simulink model "Casc_Filter_x4"  (Simulink 6.4)
settings: Solver=ode45  StartTime=0.0  StopTime=4100/sampling_freq  RelTol=1e-3
undefined symbols (not defined in the file): A, B, filter_clk, Fs, get, h_g, h_k, PCIN, sampling_freq
libraries: xbsIndex_r4 x851, dspsnks4 x9, simulink x2, dspsrcs4 x1
(part 1 of 8)
settings Model: LastModifiedBy=tbrimeye

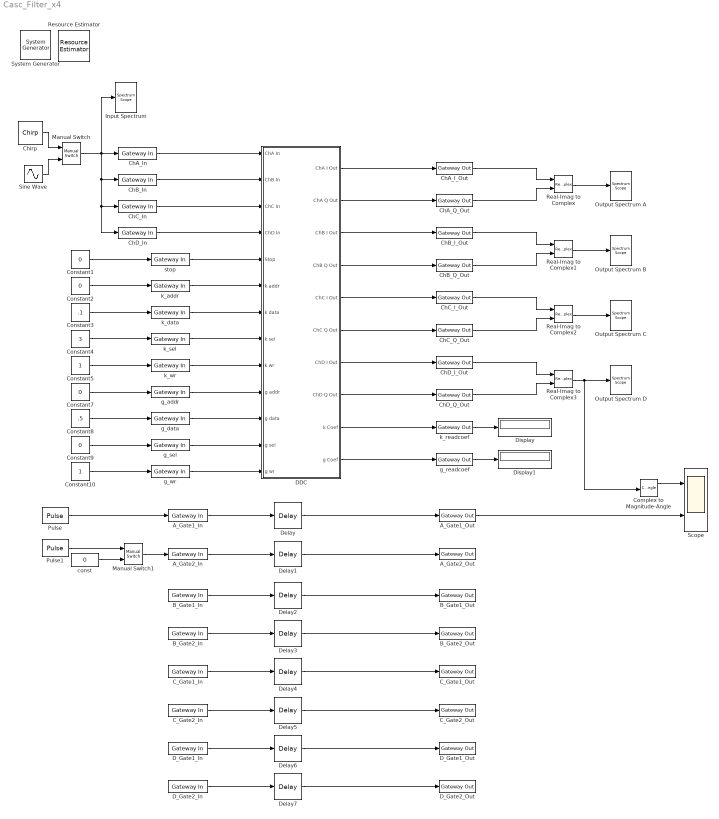
== system Casc_Filter_x4 ==
  " System Generator" : xbsIndex_r4/ System Generator  Tag=genX  SystemSampleTime=-1  xilinxfamily=Virtex4  part=xc4vsx35  speed=-11  package=ff668  synthesis_tool=XST  directory=C:/Work_Projects/Xilinx/SysGen_Outputs/DDC_Filters/Casc_Filter_x4_netlist  testbench=off  simulink_period=1/filter_clk  sysclk_period=(1/filter_clk)*1e9  incr_netlist=off  trim_vbits=Everywhere in SubSystem  dbl_ovrd=According to Block Masks  core_generation=According to Block Masks  run_coregen=off  deprecated_control=off  eval_field=0  block_type=sysgen
      settings: block_version=8.2
  A_Gate1_In : xbsIndex_r4/Gateway In  arith_type=Boolean  n_bits=18  bin_pt=0  quantization="Round  (unbiased: +/- Inf)"  overflow=Flag as error  period=1/12e6  dbl_ovrd=off  timing_constraint=None  locs_specified=off  LOCs={}  block_type=gatewayin
      settings: infoedit="Gateway in block.  Converts inputs of type Simulink integer, double and fixed point to  Xilinx fixed point type.<P><P>Hardware notes:  In hardware these blocks become top level input ports."  xl_area=[0 0 0 0 1 0 0]  block_version=8.2
  A_Gate1_Out : xbsIndex_r4/Gateway Out  hdl_port=on  timing_constraint=None  locs_specified=off  LOCs={}  block_type=gatewayout
      settings: infoedit="Gateway out block.  Converts Xilinx fixed point inputs into ouputs of type Simulink integer, double, or fixed point.<P><P>Hardware notes:  In hardware these blocks become top level output ports or are discarded, depending on how they are configured."  xl_area=[0 0 0 0 18 0 0]  block_version=VER_STRING_GOES_HERE
  A_Gate2_In : xbsIndex_r4/Gateway In  arith_type=Boolean  n_bits=18  bin_pt=0  quantization="Round  (unbiased: +/- Inf)"  overflow=Flag as error  period=1/12e6  dbl_ovrd=off  timing_constraint=None  locs_specified=off  LOCs={}  block_type=gatewayin
      settings: infoedit="Gateway in block.  Converts inputs of type Simulink integer, double and fixed point to  Xilinx fixed point type.<P><P>Hardware notes:  In hardware these blocks become top level input ports."  xl_area=[0 0 0 0 1 0 0]  block_version=8.2
  A_Gate2_Out : xbsIndex_r4/Gateway Out  hdl_port=on  timing_constraint=None  locs_specified=off  LOCs={}  block_type=gatewayout
      settings: infoedit="Gateway out block.  Converts Xilinx fixed point inputs into ouputs of type Simulink integer, double, or fixed point.<P><P>Hardware notes:  In hardware these blocks become top level output ports or are discarded, depending on how they are configured."  xl_area=[0 0 0 0 18 0 0]  block_version=VER_STRING_GOES_HERE
  B_Gate1_In : xbsIndex_r4/Gateway In  arith_type=Boolean  n_bits=18  bin_pt=0  quantization="Round  (unbiased: +/- Inf)"  overflow=Flag as error  period=1/12e6  dbl_ovrd=off  timing_constraint=None  locs_specified=off  LOCs={}  block_type=gatewayin
      settings: infoedit="Gateway in block.  Converts inputs of type Simulink integer, double and fixed point to  Xilinx fixed point type.<P><P>Hardware notes:  In hardware these blocks become top level input ports."  xl_area=[0 0 0 0 1 0 0]  block_version=8.2
  B_Gate1_Out : xbsIndex_r4/Gateway Out  hdl_port=on  timing_constraint=None  locs_specified=off  LOCs={}  block_type=gatewayout
      settings: infoedit="Gateway out block.  Converts Xilinx fixed point inputs into ouputs of type Simulink integer, double, or fixed point.<P><P>Hardware notes:  In hardware these blocks become top level output ports or are discarded, depending on how they are configured."  xl_area=[0 0 0 0 18 0 0]  block_version=VER_STRING_GOES_HERE
  B_Gate2_In : xbsIndex_r4/Gateway In  arith_type=Boolean  n_bits=18  bin_pt=0  quantization="Round  (unbiased: +/- Inf)"  overflow=Flag as error  period=1/12e6  dbl_ovrd=off  timing_constraint=None  locs_specified=off  LOCs={}  block_type=gatewayin
      settings: infoedit="Gateway in block.  Converts inputs of type Simulink integer, double and fixed point to  Xilinx fixed point type.<P><P>Hardware notes:  In hardware these blocks become top level input ports."  xl_area=[0 0 0 0 1 0 0]  block_version=8.2
  B_Gate2_Out : xbsIndex_r4/Gateway Out  hdl_port=on  timing_constraint=None  locs_specified=off  LOCs={}  block_type=gatewayout
      settings: infoedit="Gateway out block.  Converts Xilinx fixed point inputs into ouputs of type Simulink integer, double, or fixed point.<P><P>Hardware notes:  In hardware these blocks become top level output ports or are discarded, depending on how they are configured."  xl_area=[0 0 0 0 18 0 0]  block_version=VER_STRING_GOES_HERE
  C_Gate1_In : xbsIndex_r4/Gateway In  arith_type=Boolean  n_bits=18  bin_pt=0  quantization="Round  (unbiased: +/- Inf)"  overflow=Flag as error  period=1/12e6  dbl_ovrd=off  timing_constraint=None  locs_specified=off  LOCs={}  block_type=gatewayin
      settings: infoedit="Gateway in block.  Converts inputs of type Simulink integer, double and fixed point to  Xilinx fixed point type.<P><P>Hardware notes:  In hardware these blocks become top level input ports."  xl_area=[0 0 0 0 1 0 0]  block_version=8.2
  C_Gate1_Out : xbsIndex_r4/Gateway Out  hdl_port=on  timing_constraint=None  locs_specified=off  LOCs={}  block_type=gatewayout
      settings: infoedit="Gateway out block.  Converts Xilinx fixed point inputs into ouputs of type Simulink integer, double, or fixed point.<P><P>Hardware notes:  In hardware these blocks become top level output ports or are discarded, depending on how they are configured."  xl_area=[0 0 0 0 18 0 0]  block_version=VER_STRING_GOES_HERE
  C_Gate2_In : xbsIndex_r4/Gateway In  arith_type=Boolean  n_bits=18  bin_pt=0  quantization="Round  (unbiased: +/- Inf)"  overflow=Flag as error  period=1/12e6  dbl_ovrd=off  timing_constraint=None  locs_specified=off  LOCs={}  block_type=gatewayin
      settings: infoedit="Gateway in block.  Converts inputs of type Simulink integer, double and fixed point to  Xilinx fixed point type.<P><P>Hardware notes:  In hardware these blocks become top level input ports."  xl_area=[0 0 0 0 1 0 0]  block_version=8.2
  C_Gate2_Out : xbsIndex_r4/Gateway Out  hdl_port=on  timing_constraint=None  locs_specified=off  LOCs={}  block_type=gatewayout
      settings: infoedit="Gateway out block.  Converts Xilinx fixed point inputs into ouputs of type Simulink integer, double, or fixed point.<P><P>Hardware notes:  In hardware these blocks become top level output ports or are discarded, depending on how they are configured."  xl_area=[0 0 0 0 18 0 0]  block_version=VER_STRING_GOES_HERE
  ChA_I_Out : xbsIndex_r4/Gateway Out  hdl_port=on  timing_constraint=None  locs_specified=off  LOCs={}  block_type=gatewayout
      settings: infoedit="Gateway out block.  Converts Xilinx fixed point inputs into ouputs of type Simulink integer, double, or fixed point.<P><P>Hardware notes:  In hardware these blocks become top level output ports or are discarded, depending on how they are configured."  xl_area=[0 0 0 0 16 0 0]  block_version=8.2
  ChA_In : xbsIndex_r4/Gateway In  arith_type="Signed  (2's comp)"  n_bits=14  bin_pt=13  quantization="Round  (unbiased: +/- Inf)"  overflow=Saturate  period=1/sampling_freq  dbl_ovrd=off  timing_constraint=None  locs_specified=off  LOCs={}  block_type=gatewayin
      settings: infoedit="Gateway in block.  Converts inputs of type Simulink integer, double and fixed point to  Xilinx fixed point type.<P><P>Hardware notes:  In hardware these blocks become top level input ports."  xl_area=[0 0 0 0 14 0 0]  block_version=8.2
  ChA_Q_Out : xbsIndex_r4/Gateway Out  hdl_port=on  timing_constraint=None  locs_specified=off  LOCs={}  block_type=gatewayout
      settings: infoedit="Gateway out block.  Converts Xilinx fixed point inputs into ouputs of type Simulink integer, double, or fixed point.<P><P>Hardware notes:  In hardware these blocks become top level output ports or are discarded, depending on how they are configured."  xl_area=[0 0 0 0 16 0 0]  block_version=8.2
  ChB_I_Out : xbsIndex_r4/Gateway Out  hdl_port=on  timing_constraint=None  locs_specified=off  LOCs={}  block_type=gatewayout
      settings: infoedit="Gateway out block.  Converts Xilinx fixed point inputs into ouputs of type Simulink integer, double, or fixed point.<P><P>Hardware notes:  In hardware these blocks become top level output ports or are discarded, depending on how they are configured."  xl_area=[0 0 0 0 16 0 0]  block_version=8.2
  ChB_In : xbsIndex_r4/Gateway In  arith_type="Signed  (2's comp)"  n_bits=14  bin_pt=13  quantization="Round  (unbiased: +/- Inf)"  overflow=Saturate  period=1/sampling_freq  dbl_ovrd=off  timing_constraint=None  locs_specified=off  LOCs={}  block_type=gatewayin
      settings: infoedit="Gateway in block.  Converts inputs of type Simulink integer, double and fixed point to  Xilinx fixed point type.<P><P>Hardware notes:  In hardware these blocks become top level input ports."  xl_area=[0 0 0 0 14 0 0]  block_version=8.2
  ChB_Q_Out : xbsIndex_r4/Gateway Out  hdl_port=on  timing_constraint=None  locs_specified=off  LOCs={}  block_type=gatewayout
      settings: infoedit="Gateway out block.  Converts Xilinx fixed point inputs into ouputs of type Simulink integer, double, or fixed point.<P><P>Hardware notes:  In hardware these blocks become top level output ports or are discarded, depending on how they are configured."  xl_area=[0 0 0 0 16 0 0]  block_version=8.2
  ChC_I_Out : xbsIndex_r4/Gateway Out  hdl_port=on  timing_constraint=None  locs_specified=off  LOCs={}  block_type=gatewayout
      settings: infoedit="Gateway out block.  Converts Xilinx fixed point inputs into ouputs of type Simulink integer, double, or fixed point.<P><P>Hardware notes:  In hardware these blocks become top level output ports or are discarded, depending on how they are configured."  xl_area=[0 0 0 0 16 0 0]  block_version=8.2
  ChC_In : xbsIndex_r4/Gateway In  arith_type="Signed  (2's comp)"  n_bits=14  bin_pt=13  quantization="Round  (unbiased: +/- Inf)"  overflow=Saturate  period=1/sampling_freq  dbl_ovrd=off  timing_constraint=None  locs_specified=off  LOCs={}  block_type=gatewayin
      settings: infoedit="Gateway in block.  Converts inputs of type Simulink integer, double and fixed point to  Xilinx fixed point type.<P><P>Hardware notes:  In hardware these blocks become top level input ports."  xl_area=[0 0 0 0 14 0 0]  block_version=8.2
  ChC_Q_Out : xbsIndex_r4/Gateway Out  hdl_port=on  timing_constraint=None  locs_specified=off  LOCs={}  block_type=gatewayout
      settings: infoedit="Gateway out block.  Converts Xilinx fixed point inputs into ouputs of type Simulink integer, double, or fixed point.<P><P>Hardware notes:  In hardware these blocks become top level output ports or are discarded, depending on how they are configured."  xl_area=[0 0 0 0 16 0 0]  block_version=8.2
  ChD_I_Out : xbsIndex_r4/Gateway Out  hdl_port=on  timing_constraint=None  locs_specified=off  LOCs={}  block_type=gatewayout
      settings: infoedit="Gateway out block.  Converts Xilinx fixed point inputs into ouputs of type Simulink integer, double, or fixed point.<P><P>Hardware notes:  In hardware these blocks become top level output ports or are discarded, depending on how they are configured."  xl_area=[0 0 0 0 16 0 0]  block_version=8.2
  ChD_In : xbsIndex_r4/Gateway In  arith_type="Signed  (2's comp)"  n_bits=14  bin_pt=13  quantization="Round  (unbiased: +/- Inf)"  overflow=Saturate  period=1/sampling_freq  dbl_ovrd=off  timing_constraint=None  locs_specified=off  LOCs={}  block_type=gatewayin
      settings: infoedit="Gateway in block.  Converts inputs of type Simulink integer, double and fixed point to  Xilinx fixed point type.<P><P>Hardware notes:  In hardware these blocks become top level input ports."  xl_area=[0 0 0 0 14 0 0]  block_version=8.2
  ChD_Q_Out : xbsIndex_r4/Gateway Out  hdl_port=on  timing_constraint=None  locs_specified=off  LOCs={}  block_type=gatewayout
      settings: infoedit="Gateway out block.  Converts Xilinx fixed point inputs into ouputs of type Simulink integer, double, or fixed point.<P><P>Hardware notes:  In hardware these blocks become top level output ports or are discarded, depending on how they are configured."  xl_area=[0 0 0 0 16 0 0]  block_version=8.2
  Chirp : dspsrcs4/Chirp  sweep=Linear  mode=Unidirectional  f0=0  f1=sampling_freq_div2  t1=4096/sampling_freq  Tsweep=4096/sampling_freq  phase=pi/4  Ts=1/sampling_freq  spf=1  datatype=Double
  Complex to Magnitude-Angle : ComplexToMagnitudeAngle
  Constant{1..2,7,9} (4 alike) : Constant  Value=0  OutDataType=sfix(16)  ConRadixGroup=Use specified scaling  OutScaling=2^0  SampleTime=inf  FramePeriod=inf
  Constant10 : Constant  Value=1  OutDataType=sfix(16)  ConRadixGroup=Use specified scaling  OutScaling=2^0  SampleTime=inf  FramePeriod=inf
  Constant3 : Constant  Value=.1  OutDataType=sfix(16)  ConRadixGroup=Use specified scaling  OutScaling=2^0  SampleTime=inf  FramePeriod=inf
  Constant4 : Constant  Value=3  OutDataType=sfix(16)  ConRadixGroup=Use specified scaling  OutScaling=2^0  SampleTime=inf  FramePeriod=inf
  Constant5 : Constant  Value=1  OutDataType=sfix(16)  ConRadixGroup=Use specified scaling  OutScaling=2^0  SampleTime=inf  FramePeriod=inf
  Constant8 : Constant  Value=.5  OutDataType=sfix(16)  ConRadixGroup=Use specified scaling  OutScaling=2^0  SampleTime=inf  FramePeriod=inf
  DDC : Subsystem
  D_Gate1_In : xbsIndex_r4/Gateway In  arith_type=Boolean  n_bits=18  bin_pt=0  quantization="Round  (unbiased: +/- Inf)"  overflow=Flag as error  period=1/12e6  dbl_ovrd=off  timing_constraint=None  locs_specified=off  LOCs={}  block_type=gatewayin
      settings: infoedit="Gateway in block.  Converts inputs of type Simulink integer, double and fixed point to  Xilinx fixed point type.<P><P>Hardware notes:  In hardware these blocks become top level input ports."  xl_area=[0 0 0 0 1 0 0]  block_version=8.2
  D_Gate1_Out : xbsIndex_r4/Gateway Out  hdl_port=on  timing_constraint=None  locs_specified=off  LOCs={}  block_type=gatewayout
      settings: infoedit="Gateway out block.  Converts Xilinx fixed point inputs into ouputs of type Simulink integer, double, or fixed point.<P><P>Hardware notes:  In hardware these blocks become top level output ports or are discarded, depending on how they are configured."  xl_area=[0 0 0 0 18 0 0]  block_version=VER_STRING_GOES_HERE
  D_Gate2_In : xbsIndex_r4/Gateway In  arith_type=Boolean  n_bits=18  bin_pt=0  quantization="Round  (unbiased: +/- Inf)"  overflow=Flag as error  period=1/12e6  dbl_ovrd=off  timing_constraint=None  locs_specified=off  LOCs={}  block_type=gatewayin
      settings: infoedit="Gateway in block.  Converts inputs of type Simulink integer, double and fixed point to  Xilinx fixed point type.<P><P>Hardware notes:  In hardware these blocks become top level input ports."  xl_area=[0 0 0 0 1 0 0]  block_version=8.2
  D_Gate2_Out : xbsIndex_r4/Gateway Out  hdl_port=on  timing_constraint=None  locs_specified=off  LOCs={}  block_type=gatewayout
      settings: infoedit="Gateway out block.  Converts Xilinx fixed point inputs into ouputs of type Simulink integer, double, or fixed point.<P><P>Hardware notes:  In hardware these blocks become top level output ports or are discarded, depending on how they are configured."  xl_area=[0 0 0 0 18 0 0]  block_version=VER_STRING_GOES_HERE
  Delay{,1..7} (8 alike) : xbsIndex_r4/Delay  en=off  latency=9  dbl_ovrd=off  reg_retiming=off  block_type=delay
      settings: infoedit=Hardware notes: A delay line is a chain, each link of which is an SRL16 followed by a flip-flop. If register retiming is enabled, the delay line is a chain of flip-flops.  block_version=8.2
  Display : Display
  Display1 : Display
  Input Spectrum : dspsnks4/Spectrum Scope  DialogController=dspdialog.SpectrumScope  DialogControllerArgs=DataTag5  SystemSampleTime=-1  ScopeProperties=on  Domain=Frequency  HorizSpan=1  UseBuffer=on  BufferSize=4096  Overlap=64  inpFftLenInherit=on  FFTlength=4096  numAvg=2  DisplayProperties=off  AxisGrid=on  Memory=off  FrameNumber=on  AxisLegend=off  AxisZoom=off  OpenScopeAtSimStart=on  OpenScopeImmediately=off  FigPos=get(0,'defaultfigureposition')  AxisProperties=off  XUnits=Hertz  XRange=[-Fs/2...Fs/2]  InheritXIncr=on  XIncr=1.0  XLabel=Samples  YUnits=dB  YLabel=Magnitude-squared, dB  LineProperties=off  wintypeSpecScope=Boxcar  RsSpecScope=50  betaSpecScope=5  winsampSpecScope=Periodic
      settings: YMin=-100  YMax=0
  Manual Switch : simulink/Signal Routing/Manual Switch  SystemSampleTime=-1  sw=1  action=0
  Manual Switch1 : simulink/Signal Routing/Manual Switch  SystemSampleTime=-1  sw=0  action=0
  Output Spectrum A : dspsnks4/Spectrum Scope  DialogController=dspdialog.SpectrumScope  DialogControllerArgs=DataTag6  SystemSampleTime=-1  ScopeProperties=on  Domain=Frequency  HorizSpan=1  UseBuffer=on  BufferSize=1024  Overlap=64  inpFftLenInherit=on  FFTlength=1024  numAvg=2  DisplayProperties=off  AxisGrid=on  Memory=off  FrameNumber=on  AxisLegend=off  AxisZoom=off  OpenScopeAtSimStart=on  OpenScopeImmediately=off  FigPos=get(0,'defaultfigureposition')  AxisProperties=off  XUnits=Hertz  XRange=[-Fs/2...Fs/2]  InheritXIncr=on  XIncr=1.0  XLabel=Samples  YUnits=dB  YLabel=Magnitude-squared, dB  LineProperties=off  wintypeSpecScope=Boxcar  RsSpecScope=50  betaSpecScope=5  winsampSpecScope=Periodic
      settings: YMin=-120  YMax=0
  Output Spectrum B : dspsnks4/Spectrum Scope  DialogController=dspdialog.SpectrumScope  DialogControllerArgs=DataTag7  SystemSampleTime=-1  ScopeProperties=on  Domain=Frequency  HorizSpan=1  UseBuffer=on  BufferSize=1024  Overlap=64  inpFftLenInherit=on  FFTlength=1024  numAvg=2  DisplayProperties=off  AxisGrid=on  Memory=off  FrameNumber=on  AxisLegend=off  AxisZoom=off  OpenScopeAtSimStart=on  OpenScopeImmediately=off  FigPos=get(0,'defaultfigureposition')  AxisProperties=off  XUnits=Hertz  XRange=[-Fs/2...Fs/2]  InheritXIncr=on  XIncr=1.0  XLabel=Samples  YUnits=dB  YLabel=Magnitude-squared, dB  LineProperties=off  wintypeSpecScope=Boxcar  RsSpecScope=50  betaSpecScope=5  winsampSpecScope=Periodic
      settings: YMin=-120  YMax=0
  Output Spectrum C : dspsnks4/Spectrum Scope  DialogController=dspdialog.SpectrumScope  DialogControllerArgs=DataTag8  SystemSampleTime=-1  ScopeProperties=on  Domain=Frequency  HorizSpan=1  UseBuffer=on  BufferSize=1024  Overlap=64  inpFftLenInherit=on  FFTlength=1024  numAvg=2  DisplayProperties=off  AxisGrid=on  Memory=off  FrameNumber=on  AxisLegend=off  AxisZoom=off  OpenScopeAtSimStart=on  OpenScopeImmediately=off  FigPos=get(0,'defaultfigureposition')  AxisProperties=off  XUnits=Hertz  XRange=[-Fs/2...Fs/2]  InheritXIncr=on  XIncr=1.0  XLabel=Samples  YUnits=dB  YLabel=Magnitude-squared, dB  LineProperties=off  wintypeSpecScope=Boxcar  RsSpecScope=50  betaSpecScope=5  winsampSpecScope=Periodic
      settings: YMin=-120  YMax=0
  Output Spectrum D : dspsnks4/Spectrum Scope  DialogController=dspdialog.SpectrumScope  DialogControllerArgs=DataTag9  SystemSampleTime=-1  ScopeProperties=on  Domain=Frequency  HorizSpan=1  UseBuffer=on  BufferSize=1024  Overlap=64  inpFftLenInherit=on  FFTlength=1024  numAvg=2  DisplayProperties=off  AxisGrid=on  Memory=off  FrameNumber=on  AxisLegend=off  AxisZoom=off  OpenScopeAtSimStart=on  OpenScopeImmediately=off  FigPos=get(0,'defaultfigureposition')  AxisProperties=off  XUnits=Hertz  XRange=[-Fs/2...Fs/2]  InheritXIncr=on  XIncr=1.0  XLabel=Samples  YUnits=dB  YLabel=Magnitude-squared, dB  LineProperties=off  wintypeSpecScope=Boxcar  RsSpecScope=50  betaSpecScope=5  winsampSpecScope=Periodic
      settings: YMin=-120  YMax=0
  Pulse : DiscretePulseGenerator  PulseType=Time based  Period=2000/12e6  PulseWidth=50
  Pulse1 : DiscretePulseGenerator  PulseType=Time based  Period=500/12e6  PulseWidth=20
  Real-Imag to Complex{,1..3} (4 alike) : RealImagToComplex
  Resource Estimator : xbsIndex_r4/Resource Estimator  Tag=resEstTag  Slices=925  FFs=1405  BRAMs=7  LUTs=1104  IOBs=133  EBMs=14  TBUFs=0  xl_use_estimator_area=off  est_options=Post Map  xl_estimator_area=[1915 2342 0 3405 33 4 0]  block_type=resource_estimator
      settings: AttributesFormatString=Resource\nEstimator  block_version=8.2
  Scope : Scope  NumInputPorts=2
      settings: YMin=-5~-5  YMax=5~5
  Sine Wave : Sin  Frequency=2*pi*61e6  SampleTime=1/48e6
  const : Constant  Value=0  OutDataType=sfix(16)  ConRadixGroup=Use specified scaling  OutScaling=2^0  SampleTime=inf  FramePeriod=inf
  g_addr : xbsIndex_r4/Gateway In  arith_type=Unsigned  n_bits=4  bin_pt=0  quantization="Round  (unbiased: +/- Inf)"  overflow=Saturate  period=1/filter_clk  dbl_ovrd=off  timing_constraint=None  locs_specified=off  LOCs={}  block_type=gatewayin
      settings: infoedit="Gateway in block.  Converts inputs of type Simulink integer, double and fixed point to  Xilinx fixed point type.<P><P>Hardware notes:  In hardware these blocks become top level input ports."  xl_area=[0 0 0 0 4 0 0]  block_version=VER_STRING_GOES_HERE
  g_data : xbsIndex_r4/Gateway In  arith_type="Signed  (2's comp)"  n_bits=18  bin_pt=17  quantization="Round  (unbiased: +/- Inf)"  overflow=Saturate  period=1/filter_clk  dbl_ovrd=off  timing_constraint=None  locs_specified=off  LOCs={}  block_type=gatewayin
      settings: infoedit="Gateway in block.  Converts inputs of type Simulink integer, double and fixed point to  Xilinx fixed point type.<P><P>Hardware notes:  In hardware these blocks become top level input ports."  xl_area=[0 0 0 0 18 0 0]  block_version=VER_STRING_GOES_HERE
  g_readcoef : xbsIndex_r4/Gateway Out  hdl_port=on  timing_constraint=None  locs_specified=off  LOCs={}  block_type=gatewayout
      settings: infoedit="Gateway out block.  Converts Xilinx fixed point inputs into ouputs of type Simulink integer, double, or fixed point.<P><P>Hardware notes:  In hardware these blocks become top level output ports or are discarded, depending on how they are configured."  xl_area=[0 0 0 0 18 0 0]  block_version=VER_STRING_GOES_HERE
  g_sel : xbsIndex_r4/Gateway In  arith_type=Unsigned  n_bits=2  bin_pt=0  quantization="Round  (unbiased: +/- Inf)"  overflow=Saturate  period=1/filter_clk  dbl_ovrd=off  timing_constraint=None  locs_specified=off  LOCs={}  block_type=gatewayin
      settings: infoedit="Gateway in block.  Converts inputs of type Simulink integer, double and fixed point to  Xilinx fixed point type.<P><P>Hardware notes:  In hardware these blocks become top level input ports."  xl_area=[0 0 0 0 2 0 0]  block_version=VER_STRING_GOES_HERE
  g_wr : xbsIndex_r4/Gateway In  arith_type=Boolean  n_bits=4  bin_pt=0  quantization="Round  (unbiased: +/- Inf)"  overflow=Saturate  period=1/filter_clk  dbl_ovrd=off  timing_constraint=None  locs_specified=off  LOCs={}  block_type=gatewayin
      settings: infoedit="Gateway in block.  Converts inputs of type Simulink integer, double and fixed point to  Xilinx fixed point type.<P><P>Hardware notes:  In hardware these blocks become top level input ports."  xl_area=[0 0 0 0 1 0 0]  block_version=VER_STRING_GOES_HERE
  k_addr : xbsIndex_r4/Gateway In  arith_type=Unsigned  n_bits=4  bin_pt=0  quantization="Round  (unbiased: +/- Inf)"  overflow=Saturate  period=1/filter_clk  dbl_ovrd=off  timing_constraint=None  locs_specified=off  LOCs={}  block_type=gatewayin
      settings: infoedit="Gateway in block.  Converts inputs of type Simulink integer, double and fixed point to  Xilinx fixed point type.<P><P>Hardware notes:  In hardware these blocks become top level input ports."  xl_area=[0 0 0 0 4 0 0]  block_version=VER_STRING_GOES_HERE
  k_data : xbsIndex_r4/Gateway In  arith_type="Signed  (2's comp)"  n_bits=18  bin_pt=17  quantization="Round  (unbiased: +/- Inf)"  overflow=Saturate  period=1/filter_clk  dbl_ovrd=off  timing_constraint=None  locs_specified=off  LOCs={}  block_type=gatewayin
      settings: infoedit="Gateway in block.  Converts inputs of type Simulink integer, double and fixed point to  Xilinx fixed point type.<P><P>Hardware notes:  In hardware these blocks become top level input ports."  xl_area=[0 0 0 0 18 0 0]  block_version=VER_STRING_GOES_HERE
  k_readcoef : xbsIndex_r4/Gateway Out  hdl_port=on  timing_constraint=None  locs_specified=off  LOCs={}  block_type=gatewayout
      settings: infoedit="Gateway out block.  Converts Xilinx fixed point inputs into ouputs of type Simulink integer, double, or fixed point.<P><P>Hardware notes:  In hardware these blocks become top level output ports or are discarded, depending on how they are configured."  xl_area=[0 0 0 0 18 0 0]  block_version=VER_STRING_GOES_HERE
  k_sel : xbsIndex_r4/Gateway In  arith_type=Unsigned  n_bits=2  bin_pt=0  quantization="Round  (unbiased: +/- Inf)"  overflow=Saturate  period=1/filter_clk  dbl_ovrd=off  timing_constraint=None  locs_specified=off  LOCs={}  block_type=gatewayin
      settings: infoedit="Gateway in block.  Converts inputs of type Simulink integer, double and fixed point to  Xilinx fixed point type.<P><P>Hardware notes:  In hardware these blocks become top level input ports."  xl_area=[0 0 0 0 2 0 0]  block_version=VER_STRING_GOES_HERE
  k_wr : xbsIndex_r4/Gateway In  arith_type=Boolean  n_bits=4  bin_pt=0  quantization="Round  (unbiased: +/- Inf)"  overflow=Saturate  period=1/filter_clk  dbl_ovrd=off  timing_constraint=None  locs_specified=off  LOCs={}  block_type=gatewayin
      settings: infoedit="Gateway in block.  Converts inputs of type Simulink integer, double and fixed point to  Xilinx fixed point type.<P><P>Hardware notes:  In hardware these blocks become top level input ports."  xl_area=[0 0 0 0 1 0 0]  block_version=VER_STRING_GOES_HERE
  stop : xbsIndex_r4/Gateway In  arith_type=Unsigned  n_bits=1  bin_pt=0  quantization="Round  (unbiased: +/- Inf)"  overflow=Saturate  period=1/filter_clk  dbl_ovrd=off  timing_constraint=None  locs_specified=off  LOCs={}  block_type=gatewayin
      settings: infoedit="Gateway in block.  Converts inputs of type Simulink integer, double and fixed point to  Xilinx fixed point type.<P><P>Hardware notes:  In hardware these blocks become top level input ports."  xl_area=[0 0 0 0 1 0 0]  block_version=VER_STRING_GOES_HERE
  wires:
  Chirp/1 -> Manual Switch/1
  Sine Wave/1 -> Manual Switch/2
  ChA_In/1 -> DDC/1(ChA In)
  Real-Imag to Complex/1 -> Output Spectrum A/1
  Manual Switch/1 -> Input Spectrum/1, ChA_In/1, ChB_In/1, ChC_In/1, ChD_In/1
  ChA_I_Out/1 -> Real-Imag to Complex/1
  ChA_Q_Out/1 -> Real-Imag to Complex/2
  k_sel/1 -> DDC/8(k sel)
  k_addr/1 -> DDC/6(k addr)
  k_data/1 -> DDC/7(k data)
  k_wr/1 -> DDC/9(k wr)
  DDC/9(k Coef) -> k_readcoef/1
  Constant1/1 -> stop/1
  Constant2/1 -> k_addr/1
  Constant3/1 -> k_data/1
  Constant4/1 -> k_sel/1
  Constant5/1 -> k_wr/1
  k_readcoef/1 -> Display/1
  g_readcoef/1 -> Display1/1
  DDC/10(g Coef) -> g_readcoef/1
  g_addr/1 -> DDC/10(g addr)
  g_data/1 -> DDC/11(g data)
  g_sel/1 -> DDC/12(g sel)
  g_wr/1 -> DDC/13(g wr)
  Constant7/1 -> g_addr/1
  Constant8/1 -> g_data/1
  Constant9/1 -> g_sel/1
  Constant10/1 -> g_wr/1
  DDC/1(ChA I Out) -> ChA_I_Out/1
  DDC/2(ChA Q Out) -> ChA_Q_Out/1
  stop/1 -> DDC/5(Stop)
  Complex to Magnitude-Angle/1 -> Scope/1
  Pulse/1 -> A_Gate1_In/1
  Pulse1/1 -> Manual Switch1/1
  const/1 -> Manual Switch1/2
  Manual Switch1/1 -> A_Gate2_In/1
  A_Gate1_In/1 -> Delay/1
  A_Gate2_In/1 -> Delay1/1
  Delay/1 -> A_Gate1_Out/1
  Delay1/1 -> A_Gate2_Out/1
  A_Gate1_Out/1 -> Scope/2
  Real-Imag to Complex1/1 -> Output Spectrum B/1
  ChB_I_Out/1 -> Real-Imag to Complex1/1
  ChB_Q_Out/1 -> Real-Imag to Complex1/2
  DDC/3(ChB I Out) -> ChB_I_Out/1
  DDC/4(ChB Q Out) -> ChB_Q_Out/1
  Real-Imag to Complex2/1 -> Output Spectrum C/1
  ChC_I_Out/1 -> Real-Imag to Complex2/1
  ChC_Q_Out/1 -> Real-Imag to Complex2/2
  Real-Imag to Complex3/1 -> Output Spectrum D/1, Complex to Magnitude-Angle/1
  ChD_I_Out/1 -> Real-Imag to Complex3/1
  ChD_Q_Out/1 -> Real-Imag to Complex3/2
  DDC/8(ChD Q Out) -> ChD_Q_Out/1
  DDC/7(ChD I Out) -> ChD_I_Out/1
  DDC/6(ChC Q Out) -> ChC_Q_Out/1
  DDC/5(ChC I Out) -> ChC_I_Out/1
  B_Gate1_In/1 -> Delay2/1
  B_Gate2_In/1 -> Delay3/1
  Delay2/1 -> B_Gate1_Out/1
  Delay3/1 -> B_Gate2_Out/1
  C_Gate1_In/1 -> Delay4/1
  C_Gate2_In/1 -> Delay5/1
  Delay4/1 -> C_Gate1_Out/1
  Delay5/1 -> C_Gate2_Out/1
  D_Gate1_In/1 -> Delay6/1
  D_Gate2_In/1 -> Delay7/1
  Delay6/1 -> D_Gate1_Out/1
  Delay7/1 -> D_Gate2_Out/1
  ChB_In/1 -> DDC/2(ChB In)
  ChC_In/1 -> DDC/3(ChC In)
  ChD_In/1 -> DDC/4(ChD In)

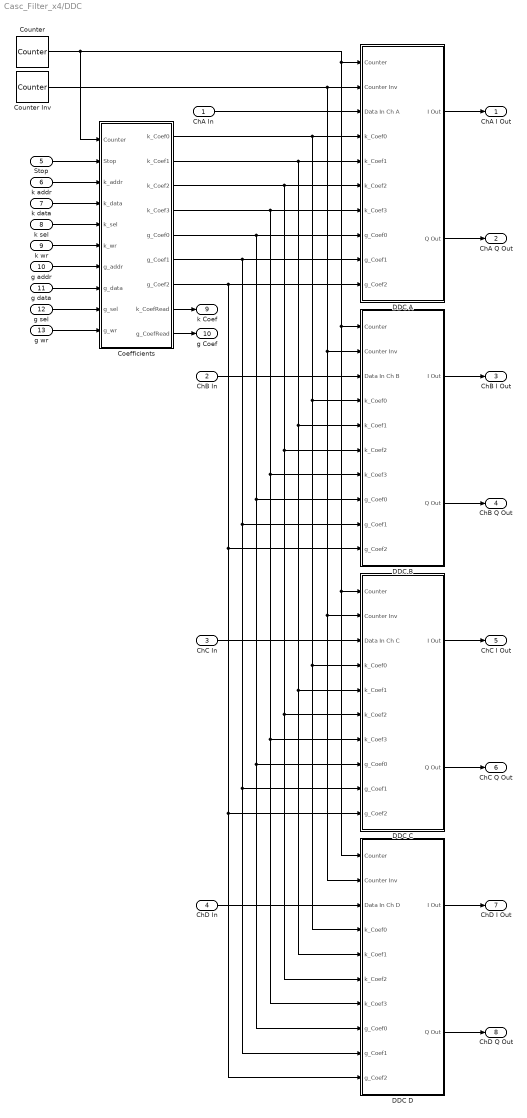
== system Casc_Filter_x4/DDC ==
  ChA In : Inport
  ChB In : Inport  Port=2
  ChC In : Inport  Port=3
  ChD In : Inport  Port=4
  Stop : Inport  Port=5
  k addr : Inport  Port=6
  k data : Inport  Port=7
  k sel : Inport  Port=8
  k wr : Inport  Port=9
  g addr : Inport  Port=10
  g data : Inport  Port=11
  g sel : Inport  Port=12
  g wr : Inport  Port=13
  Coefficients : Subsystem
  Counter : xbsIndex_r4/Counter  cnt_type=Count Limited  cnt_to=11  operation=Up  start_count=0  cnt_by_val=1  arith_type=Unsigned  n_bits=4  bin_pt=0  load_pin=off  rst=off  en=off  explicit_period=on  period=1/filter_clk  dbl_ovrd=off  use_behavioral_HDL=off  use_rpm=off  block_type=counter
      settings: block_version=8.2
  Counter Inv : xbsIndex_r4/Counter  cnt_type=Count Limited  cnt_to=0  operation=Down  start_count=11  cnt_by_val=1  arith_type=Unsigned  n_bits=4  bin_pt=0  load_pin=off  rst=off  en=off  explicit_period=on  period=1/filter_clk  dbl_ovrd=off  use_behavioral_HDL=off  use_rpm=off  block_type=counter
      settings: block_version=8.2
  DDC A : Subsystem
  DDC B : Subsystem
  DDC C : Subsystem
  DDC D : Subsystem
  ChA I Out : Outport
  ChA Q Out : Outport  Port=2
  ChB I Out : Outport  Port=3
  ChB Q Out : Outport  Port=4
  ChC I Out : Outport  Port=5
  ChC Q Out : Outport  Port=6
  ChD I Out : Outport  Port=7
  ChD Q Out : Outport  Port=8
  k Coef : Outport  Port=9
  g Coef : Outport  Port=10
  wires:
  Counter/1 -> Coefficients/1(Counter), DDC C/1(Counter), DDC D/1(Counter), DDC B/1(Counter), DDC A/1(Counter)
  Coefficients/1(k_Coef0) -> DDC C/4(k_Coef0), DDC D/4(k_Coef0), DDC B/4(k_Coef0), DDC A/4(k_Coef0)
  Coefficients/2(k_Coef1) -> DDC C/5(k_Coef1), DDC D/5(k_Coef1), DDC B/5(k_Coef1), DDC A/5(k_Coef1)
  Coefficients/3(k_Coef2) -> DDC C/6(k_Coef2), DDC D/6(k_Coef2), DDC B/6(k_Coef2), DDC A/6(k_Coef2)
  Coefficients/4(k_Coef3) -> DDC C/7(k_Coef3), DDC D/7(k_Coef3), DDC B/7(k_Coef3), DDC A/7(k_Coef3)
  Counter Inv/1 -> DDC C/2(Counter Inv), DDC D/2(Counter Inv), DDC B/2(Counter Inv), DDC A/2(Counter Inv)
  Coefficients/5(g_Coef0) -> DDC C/8(g_Coef0), DDC D/8(g_Coef0), DDC B/8(g_Coef0), DDC A/8(g_Coef0)
  Coefficients/6(g_Coef1) -> DDC C/9(g_Coef1), DDC D/9(g_Coef1), DDC B/9(g_Coef1), DDC A/9(g_Coef1)
  Coefficients/7(g_Coef2) -> DDC C/10(g_Coef2), DDC D/10(g_Coef2), DDC B/10(g_Coef2), DDC A/10(g_Coef2)
  ChA In/1 -> DDC A/3(Data In Ch A)
  Stop/1 -> Coefficients/2(Stop)
  k addr/1 -> Coefficients/3(k_addr)
  k data/1 -> Coefficients/4(k_data)
  k sel/1 -> Coefficients/5(k_sel)
  k wr/1 -> Coefficients/6(k_wr)
  g addr/1 -> Coefficients/7(g_addr)
  g data/1 -> Coefficients/8(g_data)
  Coefficients/8(k_CoefRead) -> k Coef/1
  g sel/1 -> Coefficients/9(g_sel)
  g wr/1 -> Coefficients/10(g_wr)
  Coefficients/9(g_CoefRead) -> g Coef/1
  DDC A/1(I Out) -> ChA I Out/1
  DDC A/2(Q Out) -> ChA Q Out/1
  DDC B/1(I Out) -> ChB I Out/1
  DDC B/2(Q Out) -> ChB Q Out/1
  DDC C/1(I Out) -> ChC I Out/1
  DDC C/2(Q Out) -> ChC Q Out/1
  DDC D/1(I Out) -> ChD I Out/1
  DDC D/2(Q Out) -> ChD Q Out/1
  ChB In/1 -> DDC B/3(Data In Ch B)
  ChC In/1 -> DDC C/3(Data In Ch C)
  ChD In/1 -> DDC D/3(Data In Ch D)

== system Casc_Filter_x4/DDC/Coefficients ==
  Counter : Inport
  Stop : Inport  Port=2
  k_addr : Inport  Port=3
  k_data : Inport  Port=4
  k_sel : Inport  Port=5
  k_wr : Inport  Port=6
  g_addr : Inport  Port=7
  g_data : Inport  Port=8
  g_sel : Inport  Port=9
  g_wr : Inport  Port=10
  Gaus Coef Mem : Subsystem
  Poly Coef Mem : Subsystem
  k_Coef0 : Outport
  k_Coef1 : Outport  Port=2
  k_Coef2 : Outport  Port=3
  k_Coef3 : Outport  Port=4
  g_Coef0 : Outport  Port=5
  g_Coef1 : Outport  Port=6
  g_Coef2 : Outport  Port=7
  k_CoefRead : Outport  Port=8
  g_CoefRead : Outport  Port=9
  wires:
  Stop/1 -> Gaus Coef Mem/1(Stop), Poly Coef Mem/1(Stop)
  Counter/1 -> Poly Coef Mem/2(Counter), Gaus Coef Mem/2(Counter)
  Poly Coef Mem/1(Coef0) -> k_Coef0/1
  Poly Coef Mem/2(Coef1) -> k_Coef1/1
  k_addr/1 -> Poly Coef Mem/3(Addr)
  Poly Coef Mem/3(Coef2) -> k_Coef2/1
  k_data/1 -> Poly Coef Mem/4(Data)
  Poly Coef Mem/4(Coef3) -> k_Coef3/1
  k_sel/1 -> Poly Coef Mem/5(Sel)
  Poly Coef Mem/5(Read) -> k_CoefRead/1
  k_wr/1 -> Poly Coef Mem/6(Wr/R)
  Gaus Coef Mem/1(Coef0) -> g_Coef0/1
  Gaus Coef Mem/2(Coef1) -> g_Coef1/1
  g_addr/1 -> Gaus Coef Mem/3(Addr)
  g_data/1 -> Gaus Coef Mem/4(Data)
  Gaus Coef Mem/3(Coef2) -> g_Coef2/1
  g_sel/1 -> Gaus Coef Mem/5(Sel)
  Gaus Coef Mem/4(Read) -> g_CoefRead/1
  g_wr/1 -> Gaus Coef Mem/6(Wr/R)

== system Casc_Filter_x4/DDC/DDC A ==
  Counter : Inport
  Counter Inv : Inport  Port=2
  Data In Ch A : Inport  Port=3
  k_Coef0 : Inport  Port=4
  k_Coef1 : Inport  Port=5
  k_Coef2 : Inport  Port=6
  k_Coef3 : Inport  Port=7
  g_Coef0 : Inport  Port=8
  g_Coef1 : Inport  Port=9
  g_Coef2 : Inport  Port=10
  Gateway Out : xbsIndex_r4/Gateway Out  hdl_port=off  timing_constraint=None  locs_specified=off  LOCs={}  block_type=gatewayout
      settings: infoedit="Gateway out block.  Converts Xilinx fixed point inputs into ouputs of type Simulink integer, double, or fixed point.<P><P>Hardware notes:  In hardware these blocks become top level output ports or are discarded, depending on how they are configured."  block_version=8.2
  Gateway Out1 : xbsIndex_r4/Gateway Out  hdl_port=off  timing_constraint=None  locs_specified=off  LOCs={}  block_type=gatewayout
      settings: infoedit="Gateway out block.  Converts Xilinx fixed point inputs into ouputs of type Simulink integer, double, or fixed point.<P><P>Hardware notes:  In hardware these blocks become top level output ports or are discarded, depending on how they are configured."  block_version=8.2
  Gaussian FIR Filters : Subsystem
  Poly Spectrum : dspsnks4/Spectrum Scope  DialogController=dspdialog.SpectrumScope  DialogControllerArgs=DataTag1  SystemSampleTime=-1  ScopeProperties=on  Domain=Frequency  HorizSpan=1  UseBuffer=on  BufferSize=1024  Overlap=64  inpFftLenInherit=on  FFTlength=1024  numAvg=2  DisplayProperties=off  AxisGrid=on  Memory=off  FrameNumber=on  AxisLegend=off  AxisZoom=off  OpenScopeAtSimStart=on  OpenScopeImmediately=off  FigPos=get(0,'defaultfigureposition')  AxisProperties=off  XUnits=Hertz  XRange=[-Fs/2...Fs/2]  InheritXIncr=on  XIncr=1.0  XLabel=Samples  YUnits=dB  YLabel=Magnitude-squared, dB  LineProperties=off  wintypeSpecScope=Boxcar  RsSpecScope=50  betaSpecScope=5  winsampSpecScope=Periodic
      settings: YMin=-100  YMax=0
  Polyphase Kaiser FIR Filter : Subsystem
  Real-Imag to Complex1 : RealImagToComplex
  Scope1 : Scope  NumInputPorts=2
      settings: YMin=-5~-5  YMax=5~5  SaveName=ScopeData3
  I Out : Outport
  Q Out : Outport  Port=2
  wires:
  Counter Inv/1 -> Polyphase Kaiser FIR Filter/2(Counter Inv), Gaussian FIR Filters/2(Counter Inv)
  Counter/1 -> Polyphase Kaiser FIR Filter/1(Counter), Gaussian FIR Filters/1(Counter)
  Gaussian FIR Filters/1(Q Out) -> Q Out/1
  Data In Ch A/1 -> Polyphase Kaiser FIR Filter/3(Data In)
  k_Coef0/1 -> Polyphase Kaiser FIR Filter/4(Coef0)
  Gaussian FIR Filters/2(I Out) -> I Out/1
  k_Coef1/1 -> Polyphase Kaiser FIR Filter/5(Coef1)
  k_Coef2/1 -> Polyphase Kaiser FIR Filter/6(Coef2)
  k_Coef3/1 -> Polyphase Kaiser FIR Filter/7(Coef3)
  Polyphase Kaiser FIR Filter/1(Q Out) -> Gaussian FIR Filters/3(Q In), Gateway Out1/1
  Polyphase Kaiser FIR Filter/2(I Out) -> Gaussian FIR Filters/7(I In), Gateway Out/1
  g_Coef0/1 -> Gaussian FIR Filters/4(Coef0)
  g_Coef1/1 -> Gaussian FIR Filters/5(Coef1)
  g_Coef2/1 -> Gaussian FIR Filters/6(Coef2)
  Real-Imag to Complex1/1 -> Poly Spectrum/1
  Gateway Out/1 -> Real-Imag to Complex1/1, Scope1/1
  Gateway Out1/1 -> Real-Imag to Complex1/2, Scope1/2

== system Casc_Filter_x4/DDC/DDC B ==
  Counter : Inport
  Counter Inv : Inport  Port=2
  Data In Ch B : Inport  Port=3
  k_Coef0 : Inport  Port=4
  k_Coef1 : Inport  Port=5
  k_Coef2 : Inport  Port=6
  k_Coef3 : Inport  Port=7
  g_Coef0 : Inport  Port=8
  g_Coef1 : Inport  Port=9
  g_Coef2 : Inport  Port=10
  Gateway Out : xbsIndex_r4/Gateway Out  hdl_port=off  timing_constraint=None  locs_specified=off  LOCs={}  block_type=gatewayout
      settings: infoedit="Gateway out block.  Converts Xilinx fixed point inputs into ouputs of type Simulink integer, double, or fixed point.<P><P>Hardware notes:  In hardware these blocks become top level output ports or are discarded, depending on how they are configured."  block_version=8.2
  Gateway Out1 : xbsIndex_r4/Gateway Out  hdl_port=off  timing_constraint=None  locs_specified=off  LOCs={}  block_type=gatewayout
      settings: infoedit="Gateway out block.  Converts Xilinx fixed point inputs into ouputs of type Simulink integer, double, or fixed point.<P><P>Hardware notes:  In hardware these blocks become top level output ports or are discarded, depending on how they are configured."  block_version=8.2
  Gaussian FIR Filters : Subsystem
  Poly Spectrum : dspsnks4/Spectrum Scope  DialogController=dspdialog.SpectrumScope  DialogControllerArgs=DataTag2  SystemSampleTime=-1  ScopeProperties=on  Domain=Frequency  HorizSpan=1  UseBuffer=on  BufferSize=1024  Overlap=64  inpFftLenInherit=on  FFTlength=1024  numAvg=2  DisplayProperties=off  AxisGrid=on  Memory=off  FrameNumber=on  AxisLegend=off  AxisZoom=off  OpenScopeAtSimStart=on  OpenScopeImmediately=off  FigPos=get(0,'defaultfigureposition')  AxisProperties=off  XUnits=Hertz  XRange=[-Fs/2...Fs/2]  InheritXIncr=on  XIncr=1.0  XLabel=Samples  YUnits=dB  YLabel=Magnitude-squared, dB  LineProperties=off  wintypeSpecScope=Boxcar  RsSpecScope=50  betaSpecScope=5  winsampSpecScope=Periodic
      settings: YMin=-100  YMax=0
  Polyphase Kaiser FIR Filter : Subsystem
  Real-Imag to Complex1 : RealImagToComplex
  Scope1 : Scope  NumInputPorts=2
      settings: YMin=-5~-5  YMax=5~5  SaveName=ScopeData3
  I Out : Outport
  Q Out : Outport  Port=2
  wires:
  Counter Inv/1 -> Polyphase Kaiser FIR Filter/2(Counter Inv), Gaussian FIR Filters/2(Counter Inv)
  Real-Imag to Complex1/1 -> Poly Spectrum/1
  Counter/1 -> Polyphase Kaiser FIR Filter/1(Counter), Gaussian FIR Filters/1(Counter)
  Gaussian FIR Filters/1(Q Out) -> Q Out/1
  Data In Ch B/1 -> Polyphase Kaiser FIR Filter/3(Data In)
  k_Coef0/1 -> Polyphase Kaiser FIR Filter/4(Coef0)
  Gaussian FIR Filters/2(I Out) -> I Out/1
  k_Coef1/1 -> Polyphase Kaiser FIR Filter/5(Coef1)
  k_Coef2/1 -> Polyphase Kaiser FIR Filter/6(Coef2)
  k_Coef3/1 -> Polyphase Kaiser FIR Filter/7(Coef3)
  Polyphase Kaiser FIR Filter/1(Q Out) -> Gaussian FIR Filters/3(Q In), Gateway Out1/1
  Polyphase Kaiser FIR Filter/2(I Out) -> Gaussian FIR Filters/7(I In), Gateway Out/1
  g_Coef0/1 -> Gaussian FIR Filters/4(Coef0)
  g_Coef1/1 -> Gaussian FIR Filters/5(Coef1)
  g_Coef2/1 -> Gaussian FIR Filters/6(Coef2)
  Gateway Out/1 -> Real-Imag to Complex1/1, Scope1/1
  Gateway Out1/1 -> Real-Imag to Complex1/2, Scope1/2

== system Casc_Filter_x4/DDC/DDC C ==
  Counter : Inport
  Counter Inv : Inport  Port=2
  Data In Ch C : Inport  Port=3
  k_Coef0 : Inport  Port=4
  k_Coef1 : Inport  Port=5
  k_Coef2 : Inport  Port=6
  k_Coef3 : Inport  Port=7
  g_Coef0 : Inport  Port=8
  g_Coef1 : Inport  Port=9
  g_Coef2 : Inport  Port=10
  Gateway Out : xbsIndex_r4/Gateway Out  hdl_port=off  timing_constraint=None  locs_specified=off  LOCs={}  block_type=gatewayout
      settings: infoedit="Gateway out block.  Converts Xilinx fixed point inputs into ouputs of type Simulink integer, double, or fixed point.<P><P>Hardware notes:  In hardware these blocks become top level output ports or are discarded, depending on how they are configured."  block_version=8.2
  Gateway Out1 : xbsIndex_r4/Gateway Out  hdl_port=off  timing_constraint=None  locs_specified=off  LOCs={}  block_type=gatewayout
      settings: infoedit="Gateway out block.  Converts Xilinx fixed point inputs into ouputs of type Simulink integer, double, or fixed point.<P><P>Hardware notes:  In hardware these blocks become top level output ports or are discarded, depending on how they are configured."  block_version=8.2
  Gaussian FIR Filters : Subsystem
  Poly Spectrum : dspsnks4/Spectrum Scope  DialogController=dspdialog.SpectrumScope  DialogControllerArgs=DataTag3  SystemSampleTime=-1  ScopeProperties=on  Domain=Frequency  HorizSpan=1  UseBuffer=on  BufferSize=1024  Overlap=64  inpFftLenInherit=on  FFTlength=1024  numAvg=2  DisplayProperties=off  AxisGrid=on  Memory=off  FrameNumber=on  AxisLegend=off  AxisZoom=off  OpenScopeAtSimStart=on  OpenScopeImmediately=off  FigPos=get(0,'defaultfigureposition')  AxisProperties=off  XUnits=Hertz  XRange=[-Fs/2...Fs/2]  InheritXIncr=on  XIncr=1.0  XLabel=Samples  YUnits=dB  YLabel=Magnitude-squared, dB  LineProperties=off  wintypeSpecScope=Boxcar  RsSpecScope=50  betaSpecScope=5  winsampSpecScope=Periodic
      settings: YMin=-100  YMax=0
  Polyphase Kaiser FIR Filter : Subsystem
  Real-Imag to Complex1 : RealImagToComplex
  Scope1 : Scope  NumInputPorts=2
      settings: YMin=-5~-5  YMax=5~5  SaveName=ScopeData3
  I Out : Outport
  Q Out : Outport  Port=2
  wires:
  Counter Inv/1 -> Polyphase Kaiser FIR Filter/2(Counter Inv), Gaussian FIR Filters/2(Counter Inv)
  Real-Imag to Complex1/1 -> Poly Spectrum/1
  Counter/1 -> Polyphase Kaiser FIR Filter/1(Counter), Gaussian FIR Filters/1(Counter)
  Gaussian FIR Filters/1(Q Out) -> Q Out/1
  Data In Ch C/1 -> Polyphase Kaiser FIR Filter/3(Data In)
  k_Coef0/1 -> Polyphase Kaiser FIR Filter/4(Coef0)
  Gaussian FIR Filters/2(I Out) -> I Out/1
  k_Coef1/1 -> Polyphase Kaiser FIR Filter/5(Coef1)
  k_Coef2/1 -> Polyphase Kaiser FIR Filter/6(Coef2)
  k_Coef3/1 -> Polyphase Kaiser FIR Filter/7(Coef3)
  Polyphase Kaiser FIR Filter/1(Q Out) -> Gaussian FIR Filters/3(Q In), Gateway Out1/1
  Polyphase Kaiser FIR Filter/2(I Out) -> Gaussian FIR Filters/7(I In), Gateway Out/1
  g_Coef0/1 -> Gaussian FIR Filters/4(Coef0)
  g_Coef1/1 -> Gaussian FIR Filters/5(Coef1)
  g_Coef2/1 -> Gaussian FIR Filters/6(Coef2)
  Gateway Out/1 -> Real-Imag to Complex1/1, Scope1/1
  Gateway Out1/1 -> Real-Imag to Complex1/2, Scope1/2

== system Casc_Filter_x4/DDC/DDC D ==
  Counter : Inport
  Counter Inv : Inport  Port=2
  Data In Ch D : Inport  Port=3
  k_Coef0 : Inport  Port=4
  k_Coef1 : Inport  Port=5
  k_Coef2 : Inport  Port=6
  k_Coef3 : Inport  Port=7
  g_Coef0 : Inport  Port=8
  g_Coef1 : Inport  Port=9
  g_Coef2 : Inport  Port=10
  Gateway Out : xbsIndex_r4/Gateway Out  hdl_port=off  timing_constraint=None  locs_specified=off  LOCs={}  block_type=gatewayout
      settings: infoedit="Gateway out block.  Converts Xilinx fixed point inputs into ouputs of type Simulink integer, double, or fixed point.<P><P>Hardware notes:  In hardware these blocks become top level output ports or are discarded, depending on how they are configured."  block_version=8.2
  Gateway Out1 : xbsIndex_r4/Gateway Out  hdl_port=off  timing_constraint=None  locs_specified=off  LOCs={}  block_type=gatewayout
      settings: infoedit="Gateway out block.  Converts Xilinx fixed point inputs into ouputs of type Simulink integer, double, or fixed point.<P><P>Hardware notes:  In hardware these blocks become top level output ports or are discarded, depending on how they are configured."  block_version=8.2
  Gaussian FIR Filters : Subsystem
  Poly Spectrum : dspsnks4/Spectrum Scope  DialogController=dspdialog.SpectrumScope  DialogControllerArgs=DataTag4  SystemSampleTime=-1  ScopeProperties=on  Domain=Frequency  HorizSpan=1  UseBuffer=on  BufferSize=1024  Overlap=64  inpFftLenInherit=on  FFTlength=1024  numAvg=2  DisplayProperties=off  AxisGrid=on  Memory=off  FrameNumber=on  AxisLegend=off  AxisZoom=off  OpenScopeAtSimStart=on  OpenScopeImmediately=off  FigPos=get(0,'defaultfigureposition')  AxisProperties=off  XUnits=Hertz  XRange=[-Fs/2...Fs/2]  InheritXIncr=on  XIncr=1.0  XLabel=Samples  YUnits=dB  YLabel=Magnitude-squared, dB  LineProperties=off  wintypeSpecScope=Boxcar  RsSpecScope=50  betaSpecScope=5  winsampSpecScope=Periodic
      settings: YMin=-100  YMax=0
  Polyphase Kaiser FIR Filter : Subsystem
  Real-Imag to Complex1 : RealImagToComplex
  Scope1 : Scope  NumInputPorts=2
      settings: YMin=-5~-5  YMax=5~5  SaveName=ScopeData3
  I Out : Outport
  Q Out : Outport  Port=2
  wires:
  Counter Inv/1 -> Polyphase Kaiser FIR Filter/2(Counter Inv), Gaussian FIR Filters/2(Counter Inv)
  Real-Imag to Complex1/1 -> Poly Spectrum/1
  Counter/1 -> Polyphase Kaiser FIR Filter/1(Counter), Gaussian FIR Filters/1(Counter)
  Gaussian FIR Filters/1(Q Out) -> Q Out/1
  Data In Ch D/1 -> Polyphase Kaiser FIR Filter/3(Data In)
  k_Coef0/1 -> Polyphase Kaiser FIR Filter/4(Coef0)
  Gaussian FIR Filters/2(I Out) -> I Out/1
  k_Coef1/1 -> Polyphase Kaiser FIR Filter/5(Coef1)
  k_Coef2/1 -> Polyphase Kaiser FIR Filter/6(Coef2)
  k_Coef3/1 -> Polyphase Kaiser FIR Filter/7(Coef3)
  Polyphase Kaiser FIR Filter/1(Q Out) -> Gaussian FIR Filters/3(Q In), Gateway Out1/1
  Polyphase Kaiser FIR Filter/2(I Out) -> Gaussian FIR Filters/7(I In), Gateway Out/1
  g_Coef0/1 -> Gaussian FIR Filters/4(Coef0)
  g_Coef1/1 -> Gaussian FIR Filters/5(Coef1)
  g_Coef2/1 -> Gaussian FIR Filters/6(Coef2)
  Gateway Out/1 -> Real-Imag to Complex1/1, Scope1/1
  Gateway Out1/1 -> Real-Imag to Complex1/2, Scope1/2

== system Casc_Filter_x4/DDC/Coefficients/Gaus Coef Mem ==
  Stop : Inport
  Counter : Inport  Port=2
  Addr : Inport  Port=3
  Data : Inport  Port=4
  Sel : Inport  Port=5
  Wr/R : Inport  Port=6
  Mux : xbsIndex_r4/Mux  inputs=2  en=off  latency=1  precision=Full  arith_type=Unsigned  n_bits=16  bin_pt=14  quantization=Truncate  overflow=Wrap  dbl_ovrd=off  block_type=mux
      settings: xl_area=[2 0 0 4 0 0 0]  block_version=VER_STRING_GOES_HERE
  Mux1 : xbsIndex_r4/Mux  inputs=3  en=on  latency=1  precision=Full  arith_type=Unsigned  n_bits=16  bin_pt=14  quantization=Truncate  overflow=Wrap  dbl_ovrd=off  block_type=mux
      settings: xl_area=[18 18 0 36 0 0 0]  block_version=VER_STRING_GOES_HERE
  Select Decoder : Subsystem
  Single Port RAM : xbsIndex_r4/Single Port RAM  depth=16  initVector=[h_g(1:12),0,0,0,0]  distributed_mem=Block RAM  write_mode=No Read On Write  rst=off  init_reg=0  en=off  latency=11  dbl_ovrd=off  use_rpm=off  block_type=spram
      settings: xl_area=[18 0 0 36 0 0 0]  block_version=8.2
  Single Port RAM1 : xbsIndex_r4/Single Port RAM  depth=16  initVector=[h_g(13:24),0,0,0,0]  distributed_mem=Block RAM  write_mode=No Read On Write  rst=off  init_reg=0  en=off  latency=11  dbl_ovrd=off  use_rpm=off  block_type=spram
      settings: xl_area=[18 0 0 36 0 0 0]  block_version=8.2
  Single Port RAM2 : xbsIndex_r4/Single Port RAM  depth=16  initVector=[h_g(25:36),0,0,0,0]  distributed_mem=Block RAM  write_mode=No Read On Write  rst=off  init_reg=0  en=off  latency=11  dbl_ovrd=off  use_rpm=off  block_type=spram
      settings: xl_area=[18 0 0 36 0 0 0]  block_version=8.2
  Coef0 : Outport
  Coef1 : Outport  Port=2
  Coef2 : Outport  Port=3
  Read : Outport  Port=4
  wires:
  Data/1 -> Single Port RAM1/2, Single Port RAM2/2, Single Port RAM/2
  Single Port RAM/1 -> Mux1/2, Coef0/1
  Single Port RAM1/1 -> Mux1/3, Coef1/1
  Single Port RAM2/1 -> Mux1/4, Coef2/1
  Stop/1 -> Mux/1, Select Decoder/1(Run/Stop)
  Mux/1 -> Single Port RAM/1, Single Port RAM1/1, Single Port RAM2/1
  Mux1/1 -> Read/1
  Counter/1 -> Mux/2
  Addr/1 -> Mux/3
  Sel/1 -> Select Decoder/3(Sel), Mux1/1
  Select Decoder/2(Wr0) -> Single Port RAM/3
  Select Decoder/3(Wr1) -> Single Port RAM1/3
  Select Decoder/4(Wr2) -> Single Port RAM2/3
  Wr/R/1 -> Select Decoder/2(Wr/R)
  Select Decoder/1(R_En) -> Mux1/5
